simulink model "Simulator"  (R2025b)
settings: Solver=VariableStepAuto  StartTime=0.0  StopTime=250  RelTol=1e-3
undefined symbols (not defined in the file or in its folder): params
settings Model: LastModifiedBy=Renato Filho

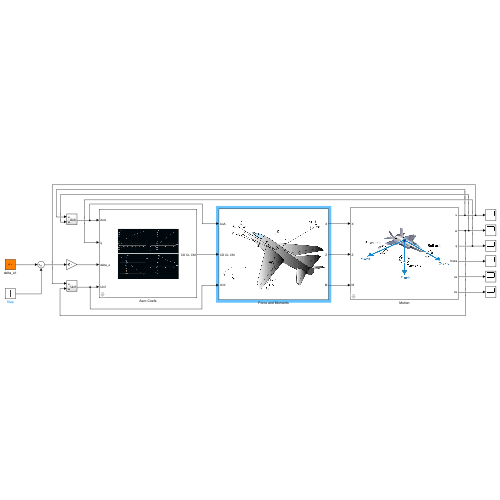
[thumbnail: Simulink's stored preview of the top-level diagram]
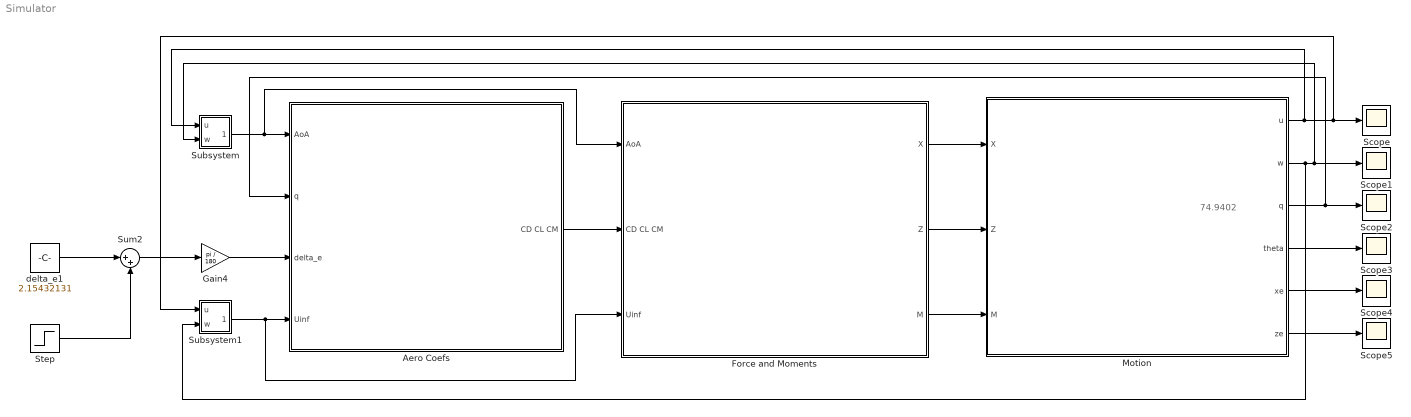
== system Simulator ==
  note: 74.9402
  Aero Coefs : Subsystem  mask{var_chord=params.chord.si}
      mask prompts: var_chord "Chord"
      mask Display: image('CDCLCM.png', [50,25,50,25,100,100]);
  Force and Moments : Subsystem
      mask Display: image('aircraft.png', [10,10,10,10,100,100]);
  Gain4 : Gain  Gain=pi / 180
  Motion : Subsystem  mask{u0=67.0860, w0=-0.2438, q0=0, theta0=-0.0036}
      mask Display: image('motion.jpg', [10,10,10,10,100,100]);
  Scope{,1..5} (6 alike) : Scope
      Scope settings: ActiveDisplayYMinimum=62.649563811287123  ActiveDisplayYMaximum=107.0139256984159  DataLoggingVariableName=uscope
      Scope1 settings: ActiveDisplayYMinimum=-4.4352547739381523  ActiveDisplayYMaximum=0.22191719710423907  DataLoggingVariableName=wscope
      Scope2 settings: ActiveDisplayYMinimum=-0.082313536113148844  ActiveDisplayYMaximum=0.033463876352101581  DataLoggingVariableName=qscope
      Scope3 settings: ActiveDisplayYMinimum=-0.3724536938312259  ActiveDisplayYMaximum=0.083961715680691468  DataLoggingVariableName=thetascope
      Scope4 settings: ActiveDisplayYMinimum=-2771.08298  ActiveDisplayYMaximum=24939.74683  DataLoggingVariableName=xescope
      Scope5 settings: ActiveDisplayYMinimum=-190.95339  ActiveDisplayYMaximum=1718.57219  DataLoggingVariableName=zescope
  Step : Step  Time=0  SampleTime=0
  Subsystem : Subsystem
  Subsystem1 : Subsystem
  Sum2 : Sum  Inputs=|++
  delta_e1 : Constant  Value=2.15432131
  wires:
  Force and Moments/1(X) -> Motion/1(X)
  Force and Moments/2(Z) -> Motion/2(Z)
  Force and Moments/3(M) -> Motion/3(M)
  Motion/4(theta) -> Scope3/1
  Motion/5(xe) -> Scope4/1
  Motion/6(ze) -> Scope5/1
  Aero Coefs/1(CD CL CM) -> Force and Moments/2(CD CL CM)
  Motion/3(q) -> Scope2/1, Aero Coefs/2(q)
  Motion/1(u) -> Subsystem/1(u), Scope/1, Subsystem1/1(u)
  Motion/2(w) -> Scope1/1, Subsystem/2(w), Subsystem1/2(w)
  Subsystem1/1(Uinf) -> Force and Moments/3(Uinf), Aero Coefs/4(Uinf)
  Subsystem/1(AoA) -> Force and Moments/1(AoA), Aero Coefs/1(AoA)
  Sum2/1 -> Gain4/1
  delta_e1/1 -> Sum2/1
  Gain4/1 -> Aero Coefs/3(delta_e)
  Step/1 -> Sum2/2

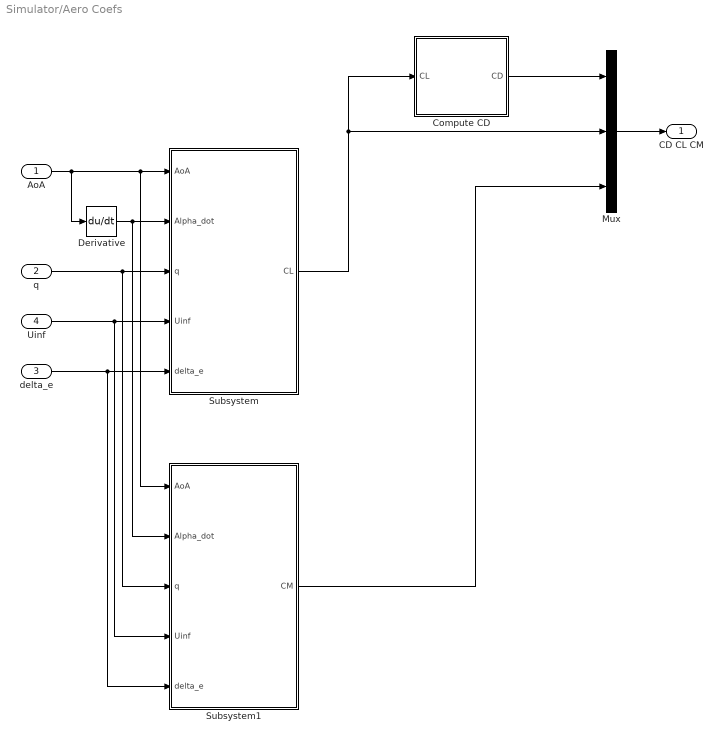
== system Simulator/Aero Coefs ==
  AoA : Inport
  q : Inport  Port=2
  delta_e : Inport  Port=3
  Uinf : Inport  Port=4
  Compute CD : Subsystem
  Derivative : Derivative
  Mux : Mux  Inputs=3
  Subsystem : Subsystem
  Subsystem1 : Subsystem
  CD CL CM : Outport
  wires:
  Subsystem1/1(CM) -> Mux/3
  Compute CD/1(CD) -> Mux/1
  Uinf/1 -> Subsystem1/4(Uinf), Subsystem/4(Uinf)
  Subsystem/1(CL) -> Mux/2, Compute CD/1(CL)
  Derivative/1 -> Subsystem1/2(Alpha_dot), Subsystem/2(Alpha_dot)
  q/1 -> Subsystem1/3(q), Subsystem/3(q)
  delta_e/1 -> Subsystem1/5(delta_e), Subsystem/5(delta_e)
  AoA/1 -> Subsystem1/1(AoA), Subsystem/1(AoA), Derivative/1
  Mux/1 -> CD CL CM/1

== system Simulator/Force and Moments ==
  AoA : Inport
  CD CL CM : Inport  Port=2
  Uinf : Inport  Port=3
  Demux : Demux  Outputs=3
  Subsystem3 : Subsystem
      mask Display: image('forces.jpg', [10,10,10,10,100,100]);
  Subsystem4 : Subsystem
      mask Display: image('xz.png');
  X : Outport
  Z : Outport  Port=2
  M : Outport  Port=3
  wires:
  Subsystem3/2(D) -> Subsystem4/3(D)
  Subsystem3/3(L) -> Subsystem4/4(L)
  Subsystem3/1(T) -> Subsystem4/2(T)
  Subsystem4/1(X) -> X/1
  AoA/1 -> Subsystem4/1(AoA)
  Demux/3 -> Subsystem3/3(CM)
  Subsystem3/4(M) -> M/1
  Uinf/1 -> Subsystem3/4(Uinf)
  Subsystem4/2(Z) -> Z/1
  CD CL CM/1 -> Demux/1
  Demux/1 -> Subsystem3/1(CD)
  Demux/2 -> Subsystem3/2(CL)

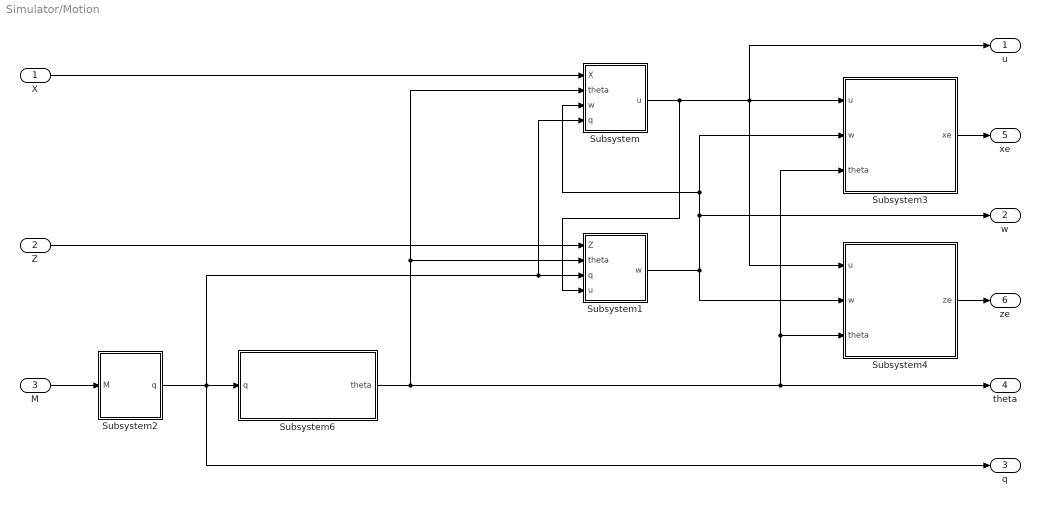
== system Simulator/Motion ==
  X : Inport
  Z : Inport  Port=2
  M : Inport  Port=3
  Subsystem : Subsystem
  Subsystem1 : Subsystem
  Subsystem2 : Subsystem
  Subsystem3 : Subsystem
  Subsystem4 : Subsystem
  Subsystem6 : Subsystem
  u : Outport
  w : Outport  Port=2
  q : Outport  Port=3
  theta : Outport  Port=4
  xe : Outport  Port=5
  ze : Outport  Port=6
  wires:
  X/1 -> Subsystem/1(X)
  Z/1 -> Subsystem1/1(Z)
  Subsystem1/1(w) -> w/1, Subsystem/3(w), Subsystem3/2(w), Subsystem4/2(w)
  Subsystem/1(u) -> Subsystem1/4(u), u/1, Subsystem4/1(u), Subsystem3/1(u)
  Subsystem6/1(theta) -> Subsystem4/3(theta), Subsystem3/3(theta), theta/1, Subsystem/2(theta), Subsystem1/2(theta)
  M/1 -> Subsystem2/1(M)
  Subsystem2/1(q) -> Subsystem6/1(q), Subsystem1/3(q), Subsystem/4(q), q/1
  Subsystem3/1(xe) -> xe/1
  Subsystem4/1(ze) -> ze/1

== system Simulator/Subsystem ==
  u : Inport
  w : Inport  Port=2
  Divide : Product  Inputs=*/
  AoA : Outport
  wires:
  Divide/1 -> AoA/1
  w/1 -> Divide/1
  u/1 -> Divide/2

== system Simulator/Subsystem1 ==
  u : Inport
  w : Inport  Port=2
  Product : Product
  Product1 : Product
  Subsystem : Subsystem
  Uinf : Outport
  wires:
  Subsystem/1(Uinf) -> Uinf/1
  Product1/1 -> Subsystem/1(u2)
  Product/1 -> Subsystem/2(w2)
  w/1 -> Product/2, Product/1
  u/1 -> Product1/2, Product1/1

== system Simulator/Aero Coefs/Compute CD ==
  CL : Inport
  CD0 : Constant  Value=params.aero.CD0
  Product : Product
  Sum : Sum
  k : Gain  Gain=params.aero.k
  CD : Outport
  wires:
  k/1 -> Sum/2
  Product/1 -> k/1
  CD0/1 -> Sum/1
  CL/1 -> Product/1, Product/2
  Sum/1 -> CD/1

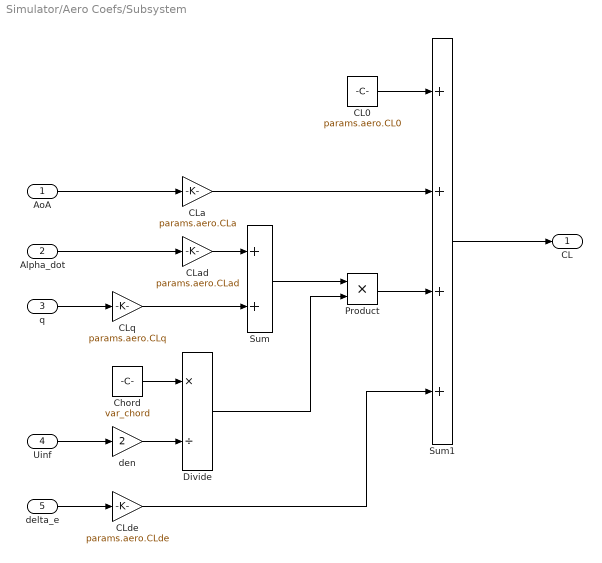
== system Simulator/Aero Coefs/Subsystem ==
  AoA : Inport
  Alpha_dot : Inport  Port=2
  q : Inport  Port=3
  Uinf : Inport  Port=4
  delta_e : Inport  Port=5
  CL0 : Constant  Value=params.aero.CL0
  CLa : Gain  Gain=params.aero.CLa
  CLad : Gain  Gain=params.aero.CLad
  CLde : Gain  Gain=params.aero.CLde
  CLq : Gain  Gain=params.aero.CLq
  Chord : Constant  Value=var_chord
  Divide : Product  Inputs=*/
  Product : Product
  Sum : Sum
  Sum1 : Sum  Inputs=++++
  den : Gain  Gain=2
  CL : Outport
  wires:
  AoA/1 -> CLa/1
  delta_e/1 -> CLde/1
  q/1 -> CLq/1
  Sum1/1 -> CL/1
  Uinf/1 -> den/1
  CL0/1 -> Sum1/1
  Chord/1 -> Divide/1
  CLde/1 -> Sum1/4
  Sum/1 -> Product/1
  Divide/1 -> Product/2
  CLa/1 -> Sum1/2
  CLad/1 -> Sum/1
  Product/1 -> Sum1/3
  Alpha_dot/1 -> CLad/1
  CLq/1 -> Sum/2
  den/1 -> Divide/2

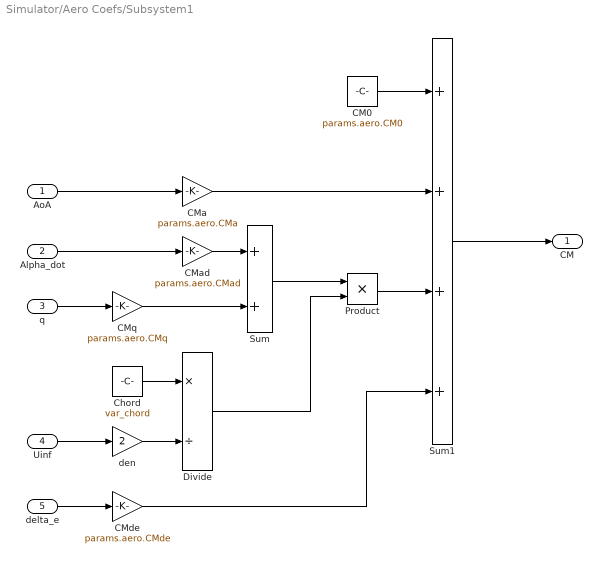
== system Simulator/Aero Coefs/Subsystem1 ==
  AoA : Inport
  Alpha_dot : Inport  Port=2
  q : Inport  Port=3
  Uinf : Inport  Port=4
  delta_e : Inport  Port=5
  CM0 : Constant  Value=params.aero.CM0
  CMa : Gain  Gain=params.aero.CMa
  CMad : Gain  Gain=params.aero.CMad
  CMde : Gain  Gain=params.aero.CMde
  CMq : Gain  Gain=params.aero.CMq
  Chord : Constant  Value=var_chord
  Divide : Product  Inputs=*/
  Product : Product
  Sum : Sum
  Sum1 : Sum  Inputs=++++
  den : Gain  Gain=2
  CM : Outport
  wires:
  AoA/1 -> CMa/1
  delta_e/1 -> CMde/1
  q/1 -> CMq/1
  Sum1/1 -> CM/1
  Uinf/1 -> den/1
  CM0/1 -> Sum1/1
  Chord/1 -> Divide/1
  CMde/1 -> Sum1/4
  Sum/1 -> Product/1
  Divide/1 -> Product/2
  CMa/1 -> Sum1/2
  CMad/1 -> Sum/1
  Product/1 -> Sum1/3
  Alpha_dot/1 -> CMad/1
  CMq/1 -> Sum/2
  den/1 -> Divide/2

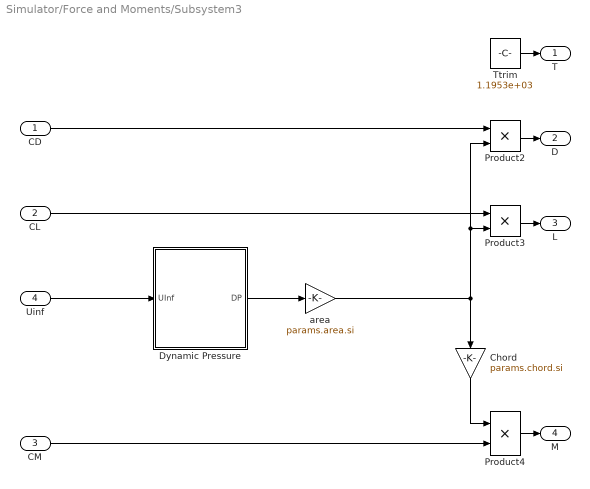
== system Simulator/Force and Moments/Subsystem3 ==
  CD : Inport
  CL : Inport  Port=2
  CM : Inport  Port=3
  Uinf : Inport  Port=4
  Chord : Gain  Gain=params.chord.si
  Dynamic Pressure : Subsystem
  Product2 : Product
  Product3 : Product
  Product4 : Product
  Ttrim : Constant  Value=1.1953e+03
  area : Gain  Gain=params.area.si
  T : Outport
  D : Outport  Port=2
  L : Outport  Port=3
  M : Outport  Port=4
  wires:
  Product2/1 -> D/1
  Product3/1 -> L/1
  CD/1 -> Product2/1
  CL/1 -> Product3/1
  Product4/1 -> M/1
  Uinf/1 -> Dynamic Pressure/1(UInf)
  CM/1 -> Product4/2
  Chord/1 -> Product4/1
  area/1 -> Product2/2, Product3/2, Chord/1
  Dynamic Pressure/1(DP) -> area/1
  Ttrim/1 -> T/1

== system Simulator/Force and Moments/Subsystem4 ==
  AoA : Inport
  T : Inport  Port=2
  D : Inport  Port=3
  L : Inport  Port=4
  Subsystem : Subsystem
  Subsystem1 : Subsystem
  X : Outport
  Z : Outport  Port=2
  wires:
  T/1 -> Subsystem/2(T), Subsystem1/2(T)
  D/1 -> Subsystem1/3(D), Subsystem/3(D)
  L/1 -> Subsystem/4(L), Subsystem1/4(L)
  AoA/1 -> Subsystem1/1(AoA), Subsystem/1(AoA)
  Subsystem/1(Z) -> Z/1
  Subsystem1/1(X) -> X/1

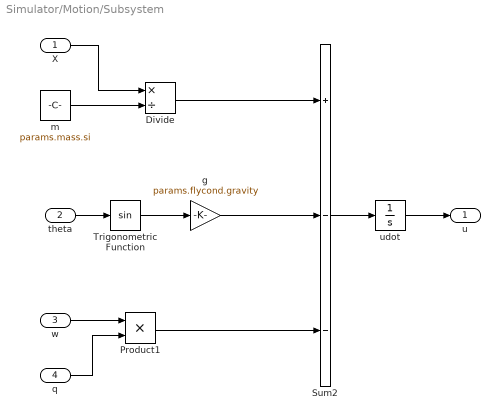
== system Simulator/Motion/Subsystem ==
  X : Inport
  theta : Inport  Port=2
  w : Inport  Port=3
  q : Inport  Port=4
  Divide : Product  Inputs=*/
  Product1 : Product
  Sum2 : Sum  Inputs=+--
  Trigonometric Function : Trigonometry
  g : Gain  Gain=params.flycond.gravity
  m : Constant  Value=params.mass.si
  udot : Integrator  InitialCondition=u0
  u : Outport
  wires:
  Divide/1 -> Sum2/1
  Trigonometric Function/1 -> g/1
  w/1 -> Product1/1
  q/1 -> Product1/2
  Product1/1 -> Sum2/3
  m/1 -> Divide/2
  g/1 -> Sum2/2
  X/1 -> Divide/1
  theta/1 -> Trigonometric Function/1
  Sum2/1 -> udot/1
  udot/1 -> u/1

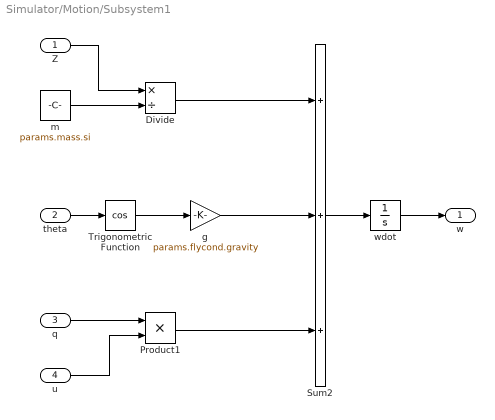
== system Simulator/Motion/Subsystem1 ==
  Z : Inport
  theta : Inport  Port=2
  q : Inport  Port=3
  u : Inport  Port=4
  Divide : Product  Inputs=*/
  Product1 : Product
  Sum2 : Sum  Inputs=+++
  Trigonometric Function : Trigonometry  Operator=cos
  g : Gain  Gain=params.flycond.gravity
  m : Constant  Value=params.mass.si
  wdot : Integrator  InitialCondition=w0
  w : Outport
  wires:
  Divide/1 -> Sum2/1
  Trigonometric Function/1 -> g/1
  q/1 -> Product1/1
  u/1 -> Product1/2
  Product1/1 -> Sum2/3
  m/1 -> Divide/2
  g/1 -> Sum2/2
  Z/1 -> Divide/1
  theta/1 -> Trigonometric Function/1
  wdot/1 -> w/1
  Sum2/1 -> wdot/1

== system Simulator/Motion/Subsystem2 ==
  M : Inport
  Divide : Product  Inputs=*/
  Iyy : Constant  Value=params.Iyy.si
  qdot : Integrator  InitialCondition=q0
  q : Outport
  wires:
  Iyy/1 -> Divide/2
  M/1 -> Divide/1
  Divide/1 -> qdot/1
  qdot/1 -> q/1

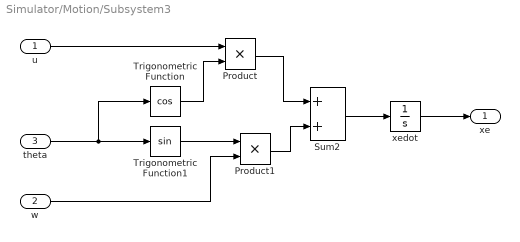
== system Simulator/Motion/Subsystem3 ==
  u : Inport
  w : Inport  Port=2
  theta : Inport  Port=3
  Product : Product
  Product1 : Product
  Sum2 : Sum
  Trigonometric Function : Trigonometry  Operator=cos
  Trigonometric Function1 : Trigonometry
  xedot : Integrator
  xe : Outport
  wires:
  xedot/1 -> xe/1
  theta/1 -> Trigonometric Function/1, Trigonometric Function1/1
  Product1/1 -> Sum2/2
  Product/1 -> Sum2/1
  Sum2/1 -> xedot/1
  u/1 -> Product/1
  Trigonometric Function/1 -> Product/2
  Trigonometric Function1/1 -> Product1/1
  w/1 -> Product1/2

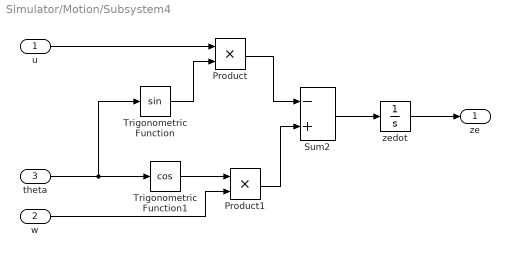
== system Simulator/Motion/Subsystem4 ==
  u : Inport
  w : Inport  Port=2
  theta : Inport  Port=3
  Product : Product
  Product1 : Product
  Sum2 : Sum  Inputs=-+
  Trigonometric Function : Trigonometry
  Trigonometric Function1 : Trigonometry  Operator=cos
  zedot : Integrator
  ze : Outport
  wires:
  zedot/1 -> ze/1
  theta/1 -> Trigonometric Function/1, Trigonometric Function1/1
  Product1/1 -> Sum2/2
  Product/1 -> Sum2/1
  Sum2/1 -> zedot/1
  u/1 -> Product/1
  Trigonometric Function/1 -> Product/2
  Trigonometric Function1/1 -> Product1/1
  w/1 -> Product1/2

== system Simulator/Motion/Subsystem6 ==
  q : Inport
  thetadot : Integrator  InitialCondition=theta0  WrapState=on  WrappedStateUpperValue=pi/2  WrappedStateLowerValue=-pi/2
  theta : Outport
  wires:
  q/1 -> thetadot/1
  thetadot/1 -> theta/1

== system Simulator/Subsystem1/Subsystem ==
  u2 : Inport
  w2 : Inport  Port=2
  Sqrt : Sqrt
  Sum : Sum
  Uinf : Outport
  wires:
  u2/1 -> Sum/1
  Sum/1 -> Sqrt/1
  w2/1 -> Sum/2
  Sqrt/1 -> Uinf/1

== system Simulator/Force and Moments/Subsystem3/Dynamic Pressure ==
  UInf : Inport
  Constant : Constant  Value=0.5
  Product : Product
  Product1 : Product  Inputs=3
  rho : Constant  Value=params.flycond.rho
  DP : Outport
  wires:
  Constant/1 -> Product1/2
  Product/1 -> Product1/1
  rho/1 -> Product1/3
  UInf/1 -> Product/2, Product/1
  Product1/1 -> DP/1

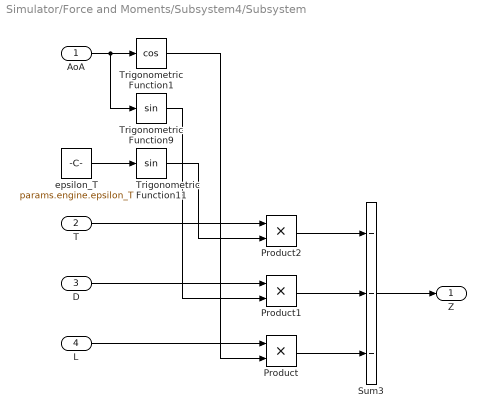
== system Simulator/Force and Moments/Subsystem4/Subsystem ==
  AoA : Inport
  T : Inport  Port=2
  D : Inport  Port=3
  L : Inport  Port=4
  Product : Product
  Product1 : Product
  Product2 : Product
  Sum3 : Sum  Inputs=---
  Trigonometric Function1 : Trigonometry  Operator=cos
  Trigonometric Function11 : Trigonometry
  Trigonometric Function9 : Trigonometry
  epsilon_T : Constant  Value=params.engine.epsilon_T
  Z : Outport
  wires:
  Sum3/1 -> Z/1
  Product/1 -> Sum3/3
  L/1 -> Product/1
  Trigonometric Function1/1 -> Product/2
  epsilon_T/1 -> Trigonometric Function11/1
  Product2/1 -> Sum3/1
  Trigonometric Function11/1 -> Product2/2
  Trigonometric Function9/1 -> Product1/2
  AoA/1 -> Trigonometric Function1/1, Trigonometric Function9/1
  Product1/1 -> Sum3/2
  D/1 -> Product1/1
  T/1 -> Product2/1

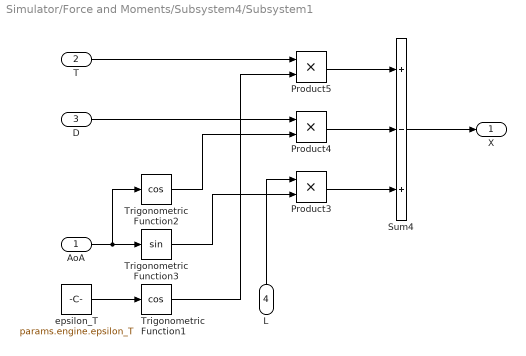
== system Simulator/Force and Moments/Subsystem4/Subsystem1 ==
  AoA : Inport
  T : Inport  Port=2
  D : Inport  Port=3
  L : Inport  Port=4
  Product3 : Product
  Product4 : Product
  Product5 : Product
  Sum4 : Sum  Inputs=+-+
  Trigonometric Function1 : Trigonometry  Operator=cos
  Trigonometric Function2 : Trigonometry  Operator=cos
  Trigonometric Function3 : Trigonometry
  epsilon_T : Constant  Value=params.engine.epsilon_T
  X : Outport
  wires:
  D/1 -> Product4/1
  Product4/1 -> Sum4/2
  epsilon_T/1 -> Trigonometric Function1/1
  Product5/1 -> Sum4/1
  Trigonometric Function1/1 -> Product5/2
  Trigonometric Function3/1 -> Product3/2
  AoA/1 -> Trigonometric Function2/1, Trigonometric Function3/1
  Sum4/1 -> X/1
  L/1 -> Product3/1
  Product3/1 -> Sum4/3
  Trigonometric Function2/1 -> Product4/2
  T/1 -> Product5/1
